simulink model "SF006A_TEstimn"  (R2013b)
settings: Solver=FixedStepDiscrete  StartTime=0.0  StopTime=1  FixedStep=0.1  RelTol=1e-3
values from neighbouring files (symbols this model uses):
  ARCHGLBPRM_100MILLISEC_SEC_F32 = DataDict.Constant    [SF006A_TEstimn_DataDict.m]
  ARCHGLBPRM_2MILLISEC_SEC_F32 = DataDict.Constant    [SF006A_TEstimn_DataDict.m]
  TEstimnAmbPwrMplr = DataDict.Calibration    [SF006A_TEstimn_DataDict.m]
  TEstimnAmbTSca = DataDict.Calibration    [SF006A_TEstimn_DataDict.m]
  TEstimnAssiMechAmbMplr = DataDict.Calibration    [SF006A_TEstimn_DataDict.m]
  TEstimnAssiMechCorrLim = DataDict.Calibration    [SF006A_TEstimn_DataDict.m]
  TEstimnAssiMechDampgSca = DataDict.Calibration    [SF006A_TEstimn_DataDict.m]
  TEstimnAssiMechDftT = DataDict.Calibration    [SF006A_TEstimn_DataDict.m]
  TEstimnAssiMechLLFilCoeffA1 = DataDict.Calibration    [SF006A_TEstimn_DataDict.m]
  TEstimnAssiMechLLFilCoeffB0 = DataDict.Calibration    [SF006A_TEstimn_DataDict.m]
  TEstimnAssiMechLLFilCoeffB1 = DataDict.Calibration    [SF006A_TEstimn_DataDict.m]
  TEstimnAssiMechSlew = DataDict.Calibration    [SF006A_TEstimn_DataDict.m]
  TESTIMNASSIMECHTHILIM_DEGCGRD_F32 = DataDict.Constant    [SF006A_TEstimn_DataDict.m]
  TESTIMNASSIMECHTLOLIM_DEGCGRD_F32 = DataDict.Constant    [SF006A_TEstimn_DataDict.m]
  TEstimnCorrnTAssiMech = DataDict.Calibration    [SF006A_TEstimn_DataDict.m]
  TEstimnCorrnTCu = DataDict.Calibration    [SF006A_TEstimn_DataDict.m]
  TEstimnCorrnTMag = DataDict.Calibration    [SF006A_TEstimn_DataDict.m]
  TEstimnCorrnTSi = DataDict.Calibration    [SF006A_TEstimn_DataDict.m]
  TEstimnCuAmbMplr = DataDict.Calibration    [SF006A_TEstimn_DataDict.m]
  TEstimnCuCorrnLim = DataDict.Calibration    [SF006A_TEstimn_DataDict.m]
  TEstimnCuLLFilCoeffA1 = DataDict.Calibration    [SF006A_TEstimn_DataDict.m]
  TEstimnCuLLFilCoeffB0 = DataDict.Calibration    [SF006A_TEstimn_DataDict.m]
  TEstimnCuLLFilCoeffB1 = DataDict.Calibration    [SF006A_TEstimn_DataDict.m]
  TEstimnEngTSca = DataDict.Calibration    [SF006A_TEstimn_DataDict.m]
  TESTIMNFETTHILIM_DEGCGRD_F32 = DataDict.Constant    [SF006A_TEstimn_DataDict.m]
  TESTIMNFETTLOLIM_DEGCGRD_F32 = DataDict.Constant    [SF006A_TEstimn_DataDict.m]
  TEstimnMagAmbMplr = DataDict.Calibration    [SF006A_TEstimn_DataDict.m]
  TEstimnMagCorrnLim = DataDict.Calibration    [SF006A_TEstimn_DataDict.m]
  TEstimnMagLLFilCoeffA1 = DataDict.Calibration    [SF006A_TEstimn_DataDict.m]
  TEstimnMagLLFilCoeffB0 = DataDict.Calibration    [SF006A_TEstimn_DataDict.m]
  TEstimnMagLLFilCoeffB1 = DataDict.Calibration    [SF006A_TEstimn_DataDict.m]
  TESTIMNMAGTHILIM_DEGCGRD_F32 = DataDict.Constant    [SF006A_TEstimn_DataDict.m]
  TESTIMNMAGTLOLIM_DEGCGRD_F32 = DataDict.Constant    [SF006A_TEstimn_DataDict.m]
  TEstimnSiAmbMplr = DataDict.Calibration    [SF006A_TEstimn_DataDict.m]
  TEstimnSiCorrnLim = DataDict.Calibration    [SF006A_TEstimn_DataDict.m]
  TEstimnSiLLFilCoeffA1 = DataDict.Calibration    [SF006A_TEstimn_DataDict.m]
  TEstimnSiLLFilCoeffB0 = DataDict.Calibration    [SF006A_TEstimn_DataDict.m]
  TEstimnSiLLFilCoeffB1 = DataDict.Calibration    [SF006A_TEstimn_DataDict.m]
  TEstimnWghtAvrgTDi = DataDict.Calibration    [SF006A_TEstimn_DataDict.m]
  TESTIMNWIDGTHILIM_DEGCGRD_F32 = DataDict.Constant    [SF006A_TEstimn_DataDict.m]
  TESTIMNWIDGTLOLIM_DEGCGRD_F32 = DataDict.Constant    [SF006A_TEstimn_DataDict.m]
undefined symbols (not defined in the file or in its folder): sigbuilder_block
libraries: NxtrLim x13, Fil x8, simulink x2
(part 2 of 3)

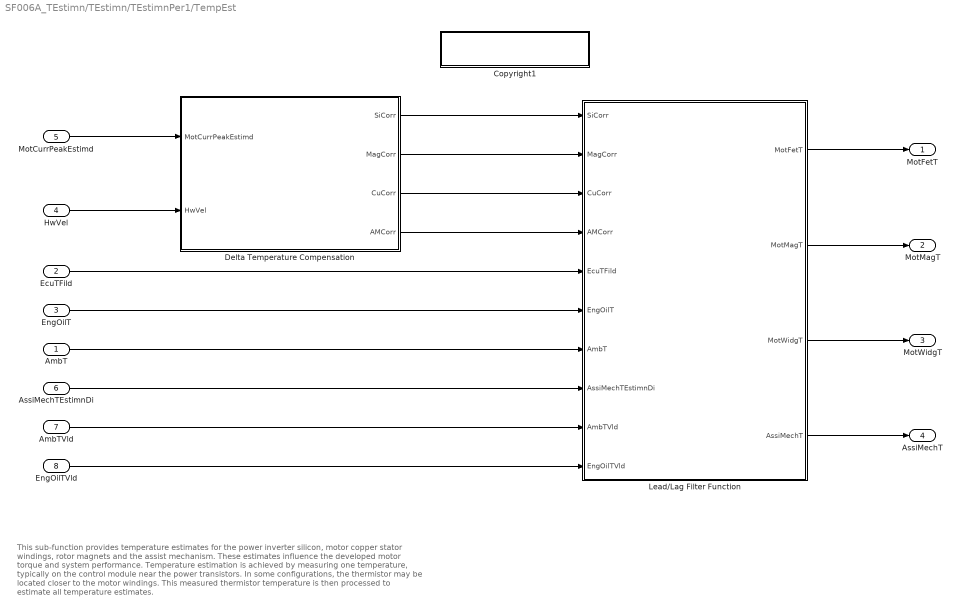
== system SF006A_TEstimn/TEstimn/TEstimnPer1/TempEst ==
  note: This sub-function provides temperature estimates for the power inverter silicon, motor copper stator windings, rotor magnets
      | and the assist mechanism. These estimates influence the developed motor torque and system performance.
      |
      | Temperature estimation is achieved by measuring one temperature, typically on the control module near the power transistors.
      | In some configurations, the thermistor may be located closer to the motor windings. This measured thermistor temperature is
      | then processed to estimate all temperature estimates.
  "AmbT " : Inport
  EcuTFild : Inport  Port=2
  "EngOilT " : Inport  Port=3
  "HwVel " : Inport  Port=4
  "MotCurrPeakEstimd " : Inport  Port=5
  AssiMechTEstimnDi : Inport  Port=6
  AmbTVld : Inport  Port=7
  EngOilTVld : Inport  Port=8
  Copyright1 : Subsystem  Description=|  RequirementInfo={} %GIDa_ed25a26e_86af_4b43_9ce6_79f2da1b6247  mask(Copyright Information){none=on}
      | Copyright info block.                                               
      |                                                                     
      | Place copyright information at the top of every subsystem in design.
      mask prompts: none "No parameters"
      mask help: Place copyright information at the top of every subsystem in design.
      mask Display:
      | NxtrConf = 'Nexteer Confidential';
      | 
      | sys = bdroot; %handle for the current model ("system")
      | first = get_param(sys,'Created');
      | if(isempty(first))
      |     first = datestr(now,'yyyy');
      | else
      |     first = first(end-3:end);  %year is last four digits
      | end
      | 
      | last = get_param(sys,'LastModifiedDate');
      | if isempty(last)
      |     last = datestr(now,'yyyy');
      | else
      |     last = last(end-3:end);
      | end
      | 
      | if strcmp(first,last)
      |     fprintf('%s\nCopyright  %s Nexteer',NxtrConf,first);
      | else
      |     fprintf('%s\n%s%s-%s Nexteer',NxtrConf,char(169),first,last);
      | end
  Delta Temperature Compensation : Subsystem  RequirementInfo={'linktype_rmi_doors' '0000a528 (/E-STEER Core/SubSystem Specifications/Application Functions/SF006A Temperature Estimation)' '#SF006A_128' 'true' 'REQ: SF006A_128' '' ; 'linktype_rmi_doors' '0000a528 (/E-STEER Core/SubSystem Specifications/Application Functions/SF006A Temperature Estimation)' '#SF006A_131' 'true' 'REQ: SF006A_131' '' ; 'linktype_rmi_doors' '0000a528 (/E-STEER Core/SubSystem Specifications/Application Functions/SF006A Temperature Estimation)' '#SF006A_145' 'true' 'REQ: SF006A_145' '' ; 'linktype_rmi_doors' '0000a528 (/E-STEER Core/SubSystem Specifications/Application Functions/SF006A Temperature Estimation)' '#SF006A_122' 'true' 'REQ: SF006A_122' '' } %GIDa_de2648f7_d571_4703_92ef_7b1b0dc2e478
  Lead/Lag Filter Function : Subsystem  RequirementInfo={'linktype_rmi_doors' '0000a528 (/E-STEER Core/SubSystem Specifications/Application Functions/SF006A Temperature Estimation)' '#SF006A_130' 'true' 'REQ: SF006A_130' '' ; 'linktype_rmi_doors' '0000a528 (/E-STEER Core/SubSystem Specifications/Application Functions/SF006A Temperature Estimation)' '#SF006A_132' 'true' 'REQ: SF006A_132' '' ; 'linktype_rmi_doors' '0000a528 (/E-STEER Core/SubSystem Specifications/Application Functions/SF006A Temperature Estimation)' '#SF006A_122' 'true' 'REQ: SF006A_122' '' ; 'linktype_rmi_doors' '0000a528 (/E-STEER Core/SubSystem Specifications/Application Functions/SF006A Temperature Estimation)' '#SF006A_170' 'true' 'REQ: SF006A_170' '' } %GIDa_ae028aaf_a7cd_4aef_92de_886aa640f764
  MotFetT : Outport
  MotMagT : Outport  Port=2
  MotWidgT : Outport  Port=3
  AssiMechT : Outport  Port=4
  wires:
  "MotCurrPeakEstimd "/1 -> Delta Temperature Compensation/1(MotCurrPeakEstimd)
  EcuTFild/1 -> Lead/Lag Filter Function/5(EcuTFild)
  Lead/Lag Filter Function/1(MotFetT) -> MotFetT/1
  Lead/Lag Filter Function/2(MotMagT) -> MotMagT/1
  Lead/Lag Filter Function/3(MotWidgT) -> MotWidgT/1
  Lead/Lag Filter Function/4(AssiMechT) -> AssiMechT/1
  "HwVel "/1 -> Delta Temperature Compensation/2(HwVel)
  "EngOilT "/1 -> Lead/Lag Filter Function/6("EngOilT ")
  "AmbT "/1 -> Lead/Lag Filter Function/7(AmbT)
  Delta Temperature Compensation/1(SiCorr) -> Lead/Lag Filter Function/1(SiCorr)
  Delta Temperature Compensation/2(MagCorr) -> Lead/Lag Filter Function/2(MagCorr)
  Delta Temperature Compensation/3(CuCorr) -> Lead/Lag Filter Function/3(CuCorr)
  Delta Temperature Compensation/4(AMCorr) -> Lead/Lag Filter Function/4(AMCorr)
  AssiMechTEstimnDi/1 -> Lead/Lag Filter Function/8(AssiMechTEstimnDi)
  EngOilTVld/1 -> Lead/Lag Filter Function/10(EngOilTVld)
  AmbTVld/1 -> Lead/Lag Filter Function/9(AmbTVld)

== system SF006A_TEstimn/TEstimn/TEstimnInit1/Assist Mechanism Temperature Initialization/AssistMechanismInitDisable ==
  EcuTFild : Inport
  Action Port : ActionPort  ActionType=else
  AssiMechT : Outport
  wires:
  EcuTFild/1 -> AssiMechT/1

== system SF006A_TEstimn/TEstimn/TEstimnInit1/Assist Mechanism Temperature Initialization/AssistMechanismInitEnable ==
  "EngOilT " : Inport
  AmbT : Inport  Port=2
  Action Port : ActionPort  ActionType=then
  Ambient Temperature Multiplier : Gain  Gain=TEstimnAmbTSca
      settings: AttributesFormatString=%<Gain>
  Engine Temperature Multiplier : Gain  Gain=TEstimnEngTSca
      settings: AttributesFormatString=%<Gain>
  Sum (4) : Sum  Inputs=+|+
  AssiMechT : Outport
  wires:
  "EngOilT "/1 -> Engine Temperature Multiplier/1
  Engine Temperature Multiplier/1 -> Sum (4)/1
  Ambient Temperature Multiplier/1 -> Sum (4)/2
  AmbT/1 -> Ambient Temperature Multiplier/1
  Sum (4)/1 -> AssiMechT/1

== system SF006A_TEstimn/TEstimn/TEstimnInit1/Assist Mechanism Temperature Initialization/Copyright1 ==

== system SF006A_TEstimn/TEstimn/TEstimnInit1/Assist Mechanism Temperature LeagLag Filter Initialization/Copyright1 ==

== system SF006A_TEstimn/TEstimn/TEstimnInit1/Motor Magnet Temperature Initialization/Copyright1 ==

== system SF006A_TEstimn/TEstimn/TEstimnInit1/Motor Magnet Temperature LeadLag Filter Initialization/Copyright1 ==

== system SF006A_TEstimn/TEstimn/TEstimnInit1/Motor Silicon Temperature Initialization/Copyright1 ==

== system SF006A_TEstimn/TEstimn/TEstimnInit1/Motor Silicon Temperature LeadLag Filter Initialization/Copyright1 ==

== system SF006A_TEstimn/TEstimn/TEstimnInit1/Motor Winding  Temperature Initialization /Copyright1 ==

== system SF006A_TEstimn/TEstimn/TEstimnInit1/Motor Winding  Temperature Lead Lag Initialization /Copyright1 ==

== system SF006A_TEstimn/TEstimn/TEstimnPer1/TempEst/Copyright1 ==

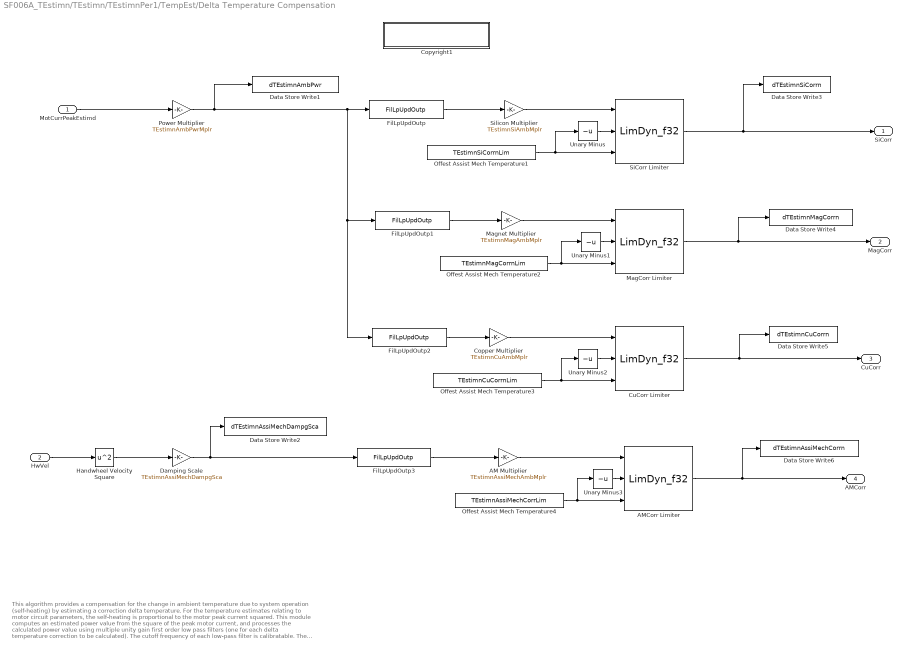
== system SF006A_TEstimn/TEstimn/TEstimnPer1/TempEst/Delta Temperature Compensation ==
  note: This algorithm provides a compensation for the change in ambient temperature due to system operation (self-heating) by estimating
      | a correction delta temperature.
      |
      | For the temperature estimates relating to motor circuit parameters, the self-heating is proportional to the motor peak current squared.
      | This module computes an estimated power value from the square of the peak motor current, and processes the calculated power value
      | using multiple unity gain first order low pass filters (one for each delta temperature correction to be calculated). The cutoff frequency of
      | each low-pass filter is calibratable. The output of each low pass filter is multiplied by a calibratable multiplier to appropriately scale the
      | result for each temperature estimate. The estimated correction temperature is also limited by a lower and upper bound.
      | For the assist mechanism temperature estimate, the self-heating is primarily due to energy dissipated due to system damping losses
      | which are proportional to the square of the rotational speed of the assist mechanism. The handwheel velocity is used to represent the
      | assist mechanism velocity. The handwheel velocity is squared and then scaled by a damping constant, and thereafter filtered through a
      | low pass filter with a calibratable frequency.
      |
      | Note that the state variables of all low pass filters must be initialized to zero at the beginning of each ignition cycle.
  MotCurrPeakEstimd : Inport
  HwVel : Inport  Port=2
  AM Multiplier : Gain  Gain=TEstimnAssiMechAmbMplr
      settings: AttributesFormatString=%<Gain>
  AMCorr Limiter : NxtrLim/LimDyn_f32
  Copper Multiplier : Gain  Gain=TEstimnCuAmbMplr
      settings: AttributesFormatString=%<Gain>
  Copyright1 : Subsystem  Description=|  RequirementInfo={} %GIDa_bd808200_6657_4ccc_9ad3_e79ac2c751ed  mask(Copyright Information){none=on}
      | Copyright info block.                                               
      |                                                                     
      | Place copyright information at the top of every subsystem in design.
      mask prompts: none "No parameters"
      mask help: Place copyright information at the top of every subsystem in design.
      mask Display:
      | NxtrConf = 'Nexteer Confidential';
      | 
      | sys = bdroot; %handle for the current model ("system")
      | first = get_param(sys,'Created');
      | if(isempty(first))
      |     first = datestr(now,'yyyy');
      | else
      |     first = first(end-3:end);  %year is last four digits
      | end
      | 
      | last = get_param(sys,'LastModifiedDate');
      | if isempty(last)
      |     last = datestr(now,'yyyy');
      | else
      |     last = last(end-3:end);
      | end
      | 
      | if strcmp(first,last)
      |     fprintf('%s\nCopyright  %s Nexteer',NxtrConf,first);
      | else
      |     fprintf('%s\n%s%s-%s Nexteer',NxtrConf,char(169),first,last);
      | end
  CuCorr Limiter : NxtrLim/LimDyn_f32
  Damping Scale : Gain  Gain=TEstimnAssiMechDampgSca  OutDataTypeStr=Inherit: Inherit via back propagation
      settings: AttributesFormatString=%<Gain>
  Data Store Write1 : DataStoreWrite  DataStoreName=dTEstimnAmbPwr
  Data Store Write2 : DataStoreWrite  DataStoreName=dTEstimnAssiMechDampgSca
  Data Store Write3 : DataStoreWrite  DataStoreName=dTEstimnSiCorrn
  Data Store Write4 : DataStoreWrite  DataStoreName=dTEstimnMagCorrn
  Data Store Write5 : DataStoreWrite  DataStoreName=dTEstimnCuCorrn
  Data Store Write6 : DataStoreWrite  DataStoreName=dTEstimnAssiMechCorrn
  FilLpUpdOutp : Fil/FilLpUpdOutp  StVar=SiFilLp
      settings: AttributesFormatString=StVar: %<StVar>
  FilLpUpdOutp1 : Fil/FilLpUpdOutp  StVar=MagFilLp
      settings: AttributesFormatString=StVar: %<StVar>
  FilLpUpdOutp2 : Fil/FilLpUpdOutp  StVar=CuFilLp
      settings: AttributesFormatString=StVar: %<StVar>
  FilLpUpdOutp3 : Fil/FilLpUpdOutp  StVar=AssiMechFilLp
      settings: AttributesFormatString=StVar: %<StVar>
  Handwheel Velocity Square : Math  Operator=square  OutDataTypeStr=Inherit: Inherit via back propagation  SaturateOnIntegerOverflow=on
  MagCorr Limiter : NxtrLim/LimDyn_f32
  Magnet Multiplier : Gain  Gain=TEstimnMagAmbMplr
      settings: AttributesFormatString=%<Gain>
  Offest Assist Mech Temperature1 : Constant  Value=TEstimnSiCorrnLim
  Offest Assist Mech Temperature2 : Constant  Value=TEstimnMagCorrnLim
  Offest Assist Mech Temperature3 : Constant  Value=TEstimnCuCorrnLim
  Offest Assist Mech Temperature4 : Constant  Value=TEstimnAssiMechCorrLim
  Power Multiplier : Gain  Gain=TEstimnAmbPwrMplr
      settings: AttributesFormatString=%<Gain>
  SiCorr Limiter : NxtrLim/LimDyn_f32
  Silicon Multiplier : Gain  Gain=TEstimnSiAmbMplr
      settings: AttributesFormatString=%<Gain>
  Unary Minus{,1..3} (4 alike) : UnaryMinus
  SiCorr : Outport
  MagCorr : Outport  Port=2
  CuCorr : Outport  Port=3
  AMCorr : Outport  Port=4
  wires:
  MotCurrPeakEstimd/1 -> Power Multiplier/1
  Silicon Multiplier/1 -> SiCorr Limiter/1
  Magnet Multiplier/1 -> MagCorr Limiter/1
  MagCorr Limiter/1 -> MagCorr/1, Data Store Write4/1
  Copper Multiplier/1 -> CuCorr Limiter/1
  AM Multiplier/1 -> AMCorr Limiter/1
  Damping Scale/1 -> Data Store Write2/1, FilLpUpdOutp3/1
  FilLpUpdOutp1/1 -> Magnet Multiplier/1
  Power Multiplier/1 -> Data Store Write1/1, FilLpUpdOutp2/1, FilLpUpdOutp1/1, FilLpUpdOutp/1
  FilLpUpdOutp/1 -> Silicon Multiplier/1
  FilLpUpdOutp2/1 -> Copper Multiplier/1
  FilLpUpdOutp3/1 -> AM Multiplier/1
  CuCorr Limiter/1 -> Data Store Write5/1, CuCorr/1
  Handwheel Velocity Square/1 -> Damping Scale/1
  HwVel/1 -> Handwheel Velocity Square/1
  Offest Assist Mech Temperature1/1 -> Unary Minus/1, SiCorr Limiter/3
  Unary Minus/1 -> SiCorr Limiter/2
  SiCorr Limiter/1 -> Data Store Write3/1, SiCorr/1
  Offest Assist Mech Temperature2/1 -> Unary Minus1/1, MagCorr Limiter/3
  Unary Minus1/1 -> MagCorr Limiter/2
  Offest Assist Mech Temperature3/1 -> Unary Minus2/1, CuCorr Limiter/3
  Unary Minus2/1 -> CuCorr Limiter/2
  Offest Assist Mech Temperature4/1 -> AMCorr Limiter/3, Unary Minus3/1
  Unary Minus3/1 -> AMCorr Limiter/2
  AMCorr Limiter/1 -> AMCorr/1, Data Store Write6/1

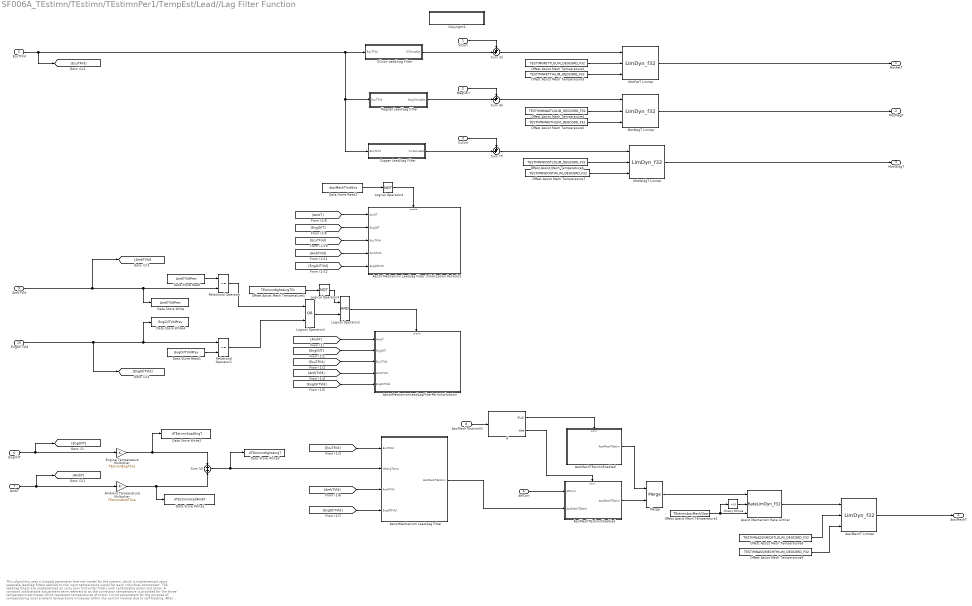
== system SF006A_TEstimn/TEstimn/TEstimnPer1/TempEst/Lead//Lag Filter Function ==
  note: This algorithm uses a lumped parameter thermal model for the system, which is implemented using separate lead/lag filters applied to the
      | input temperature signal for each individual component. The lead/lag filters are implemented as unity gain first-order filters with calibratable
      | poles and zeros.
      |
      | A constant calibratable adjustment term referred to as the correction temperature is provided for the three temperature estimates which represent
      | temperatures of motor circuit parameters for the purpose of compensating local ambient temperature increases within the control module
      | due to self-heating. After filtering the adjusted measured temperature, the corresponding correction term is added to the filter output to obtain
      | the final temperature estimate.
      | The Assist Mechanism temperature may be completely decoupled from the controller temperature and therefore the temperature estimate
      | filter does not use the measured controller temperature for an input. Two temperature inputs received from the vehicle serial communications
      | interface, namely the engine and ambient temperatures are used instead. Both of them are scaled separately and added, and this composite
      | temperature is used as the input to the lead/lag filter. Thereafter, the correction temperature is added to obtain the final estimate, and the rate
      | of change of the output is limited by a slew rate. The Assist Mechanism can be completely defeated using a serial communications message
      | if required.
      |
      | The exact details of the architecture as well as the method of initialization and reinitialization of each lead-lag flter is specified inside the
      | appropriate subsystems above.
  SiCorr : Inport
  MagCorr : Inport  Port=2
  CuCorr : Inport  Port=3
  AMCorr : Inport  Port=4
  EcuTFild : Inport  Port=5
  "EngOilT " : Inport  Port=6
  AmbT : Inport  Port=7
  AssiMechTEstimnDi : Inport  Port=8
  AmbTVld : Inport  Port=9
  EngOilTVld : Inport  Port=10
  Ambient Temperature Multiplier : Gain  Gain=TEstimnAmbTSca
      settings: AttributesFormatString=%<Gain>
  AssiMechT Limiter : NxtrLim/LimDyn_f32  RequirementInfo={'linktype_rmi_doors' '0000a528 (/E-STEER Core/SubSystem Specifications/Application Functions/SF006A Temperature Estimation)' '#SF006A_146' 'true' 'REQ: SF006A_146' '' } %GIDa_6c7b509c_1943_4e07_8eaa_8fab763417b2
  AssiMechTEstimnDisabled : Subsystem  RequirementInfo={'linktype_rmi_doors' '0000a528 (/E-STEER Core/SubSystem Specifications/Application Functions/SF006A Temperature Estimation)' '#SF006A_172' 'true' 'REQ: SF006A_172' '' } %GIDa_63efcaa1_2f18_430b_bd87_31b2ba6394f0  TreatAsAtomicUnit=on
  AssiMechTEstimnEnabled : Subsystem  RequirementInfo={'linktype_rmi_doors' '0000a528 (/E-STEER Core/SubSystem Specifications/Application Functions/SF006A Temperature Estimation)' '#SF006A_140' 'true' 'REQ: SF006A_140' '' ; 'linktype_rmi_doors' '0000a528 (/E-STEER Core/SubSystem Specifications/Application Functions/SF006A Temperature Estimation)' '#SF006A_172' 'true' 'REQ: SF006A_172' '' } %GIDa_baf7acd0_a9d7_4171_bbf7_6ce56e99201e  TreatAsAtomicUnit=on
  Assist Mechanism LeadLag Filter Initialization Periodic1 : Subsystem
  Assist Mechanism Rate Limiter : NxtrLim/RateLimDyn_f32  RequirementInfo={'linktype_rmi_doors' '0000a528 (/E-STEER Core/SubSystem Specifications/Application Functions/SF006A Temperature Estimation)' '#SF006A_159' 'true' 'REQ: SF006A_159' '' } %GIDa_cb60f311_8e3b_4de8_bd2f_2548d52e3f95  StVar=AssiMechTSlewLimPrev  Ts=ARCHGLBPRM_2MILLISEC_SEC_F32
      settings: AttributesFormatString=StVar: %<StVar>
  AssistMechanism Lead/Lag Filter : Subsystem  RequirementInfo={'linktype_rmi_doors' '0000a528 (/E-STEER Core/SubSystem Specifications/Application Functions/SF006A Temperature Estimation)' '#SF006A_135' 'true' 'REQ: SF006A_135' '' ; 'linktype_rmi_doors' '0000a528 (/E-STEER Core/SubSystem Specifications/Application Functions/SF006A Temperature Estimation)' '#SF006A_172' 'true' 'REQ: SF006A_172' '' } %GIDa_9c5c2d5a_035f_4761_9bec_ce6d38b05342
  AssistMechanismLeadLagFilterRe-Initialization : Subsystem  TreatAsAtomicUnit=on
  Copper Lead/Lag Filter : Subsystem  RequirementInfo={'linktype_rmi_doors' '0000a528 (/E-STEER Core/SubSystem Specifications/Application Functions/SF006A Temperature Estimation)' '#SF006A_171' 'true' 'REQ: SF006A_171' '' } %GIDa_b47124fe_ed06_4a6b_a9f5_ebcf66ffad42
  Copyright1 : Subsystem  Description=|  RequirementInfo={} %GIDa_98982cac_2d88_4b10_afa1_ae036335a444  mask(Copyright Information){none=on}
      | Copyright info block.                                               
      |                                                                     
      | Place copyright information at the top of every subsystem in design.
      mask prompts: none "No parameters"
      mask help: Place copyright information at the top of every subsystem in design.
      mask Display:
      | NxtrConf = 'Nexteer Confidential';
      | 
      | sys = bdroot; %handle for the current model ("system")
      | first = get_param(sys,'Created');
      | if(isempty(first))
      |     first = datestr(now,'yyyy');
      | else
      |     first = first(end-3:end);  %year is last four digits
      | end
      | 
      | last = get_param(sys,'LastModifiedDate');
      | if isempty(last)
      |     last = datestr(now,'yyyy');
      | else
      |     last = last(end-3:end);
      | end
      | 
      | if strcmp(first,last)
      |     fprintf('%s\nCopyright  %s Nexteer',NxtrConf,first);
      | else
      |     fprintf('%s\n%s%s-%s Nexteer',NxtrConf,char(169),first,last);
      | end
  Data Store Read : DataStoreRead  RequirementInfo={} %GIDa_9b0d40be_6666_4069_9c10_2ef51a624236  Priority=1  DataStoreName=AmbTVldPrev
      settings: AttributesFormatString="priority:  %<Priority>"
  Data Store Read1 : DataStoreRead  RequirementInfo={} %GIDa_19f52dbd_d2eb_4401_aae4_fbee21640a93  Priority=1  DataStoreName=EngOilTVldPrev
      settings: AttributesFormatString="priority:  %<Priority>"
  Data Store Read2 : DataStoreRead  DataStoreName=AssiMechTInitEna
  Data Store Write : DataStoreWrite  RequirementInfo={} %GIDa_1d441e6b_1fe9_4535_b703_6a16c57ac31c  Priority=2  DataStoreName=AmbTVldPrev
      settings: AttributesFormatString="priority:  %<Priority>"
  Data Store Write1 : DataStoreWrite  DataStoreName=dTEstimnScadAmbT
  Data Store Write2 : DataStoreWrite  DataStoreName=dTEstimnScadEngT
  Data Store Write3 : DataStoreWrite  DataStoreName=dTEstimnWghtAvrgT
  Data Store Write4 : DataStoreWrite  RequirementInfo={} %GIDa_a41cefac_a2e7_4b3f_b55c_d03ffcb12746  Priority=2  DataStoreName=EngOilTVldPrev
      settings: AttributesFormatString="priority:  %<Priority>"
  Engine Temperature Multiplier : Gain  Gain=TEstimnEngTSca
      settings: AttributesFormatString=%<Gain>
  If : If  IfExpression=u1
  Logical Operator1 : Logic  Operator=OR  AllPortsSameDT=off  OutDataTypeStr=boolean
  Logical Operator2 : Logic  AllPortsSameDT=off  OutDataTypeStr=boolean
  Logical Operator3 : Logic  Operator=NOT  AllPortsSameDT=off  OutDataTypeStr=boolean
  Logical Operator4 : Logic  Operator=NOT  AllPortsSameDT=off  OutDataTypeStr=boolean
  Magnet Lead/Lag Filter : Subsystem  RequirementInfo={'linktype_rmi_doors' '0000a528 (/E-STEER Core/SubSystem Specifications/Application Functions/SF006A Temperature Estimation)' '#SF006A_171' 'true' 'REQ: SF006A_171' '' } %GIDa_7145ecc5_8b30_4b7b_a3cc_c56f31d6ad47
  Merge : Merge
  MotFetT Limiter : NxtrLim/LimDyn_f32  RequirementInfo={'linktype_rmi_doors' '0000a528 (/E-STEER Core/SubSystem Specifications/Application Functions/SF006A Temperature Estimation)' '#SF006A_145' 'true' 'REQ: SF006A_145' '' ; 'linktype_rmi_doors' '0000a528 (/E-STEER Core/SubSystem Specifications/Application Functions/SF006A Temperature Estimation)' '#SF006A_147' 'true' 'REQ: SF006A_147' '' } %GIDa_13b78bce_d48c_485b_a8dd_8058a9fb1436
  MotMagT Limiter : NxtrLim/LimDyn_f32  RequirementInfo={'linktype_rmi_doors' '0000a528 (/E-STEER Core/SubSystem Specifications/Application Functions/SF006A Temperature Estimation)' '#SF006A_145' 'true' 'REQ: SF006A_145' '' ; 'linktype_rmi_doors' '0000a528 (/E-STEER Core/SubSystem Specifications/Application Functions/SF006A Temperature Estimation)' '#SF006A_147' 'true' 'REQ: SF006A_147' '' } %GIDa_60e1fd0e_a47d_43d3_86eb_3d2e6fed4866
  MotWidgT Limiter : NxtrLim/LimDyn_f32  RequirementInfo={'linktype_rmi_doors' '0000a528 (/E-STEER Core/SubSystem Specifications/Application Functions/SF006A Temperature Estimation)' '#SF006A_145' 'true' 'REQ: SF006A_145' '' ; 'linktype_rmi_doors' '0000a528 (/E-STEER Core/SubSystem Specifications/Application Functions/SF006A Temperature Estimation)' '#SF006A_147' 'true' 'REQ: SF006A_147' '' } %GIDa_2ee89f54_1f0f_4cc5_a14a_4440940f8ffc
  Offest Assist Mech Temperature1 : Constant  Value=TEstimnAssiMechSlew
  Offest Assist Mech Temperature2 : Constant  Value=TESTIMNFETTLOLIM_DEGCGRD_F32
  Offest Assist Mech Temperature3 : Constant  Value=TESTIMNFETTHILIM_DEGCGRD_F32
  Offest Assist Mech Temperature4 : Constant  Value=TESTIMNMAGTLOLIM_DEGCGRD_F32
  Offest Assist Mech Temperature5 : Constant  Value=TESTIMNMAGTHILIM_DEGCGRD_F32
  Offest Assist Mech Temperature6 : Constant  Value=TESTIMNWIDGTLOLIM_DEGCGRD_F32
  Offest Assist Mech Temperature7 : Constant  Value=TESTIMNWIDGTHILIM_DEGCGRD_F32
  Offest Assist Mech Temperature8 : Constant  Value=TESTIMNASSIMECHTLOLIM_DEGCGRD_F32
  Offest Assist Mech Temperature9 : Constant  Value=TESTIMNASSIMECHTHILIM_DEGCGRD_F32
  Offset Assist Mech Temperature1 : Constant  Value=TEstimnWghtAvrgTDi
  Relational Operator : RelationalOperator  Operator=~=  OutDataTypeStr=boolean
  Relational Operator1 : RelationalOperator  Operator=~=  OutDataTypeStr=boolean
  Silicon Lead/Lag Filter : Subsystem  RequirementInfo={'linktype_rmi_doors' '0000a528 (/E-STEER Core/SubSystem Specifications/Application Functions/SF006A Temperature Estimation)' '#SF006A_171' 'true' 'REQ: SF006A_171' '' } %GIDa_b6608b44_3176_48f0_b014_86631610bce1
  Sum (4) : Sum  Inputs=+|+
  Sum (5) : Sum  Inputs=++|
  Sum (6) : Sum  Inputs=++|
  Sum (7) : Sum  Inputs=++|
  Unary Minus : UnaryMinus
  MotFetT : Outport
  MotMagT : Outport  Port=2
  MotWidgT : Outport  Port=3
  AssiMechT : Outport  Port=4
  wires:
  EcuTFild/1 -> [EcuTFild], Silicon Lead/Lag Filter/1(EcuTFild), Copper Lead/Lag Filter/1(EcuTFild), Magnet Lead/Lag Filter/1(EcuTFild)
  MagCorr/1 -> Sum (6)/1
  CuCorr/1 -> Sum (7)/1
  SiCorr/1 -> Sum (5)/1
  Engine Temperature Multiplier/1 -> Sum (4)/1, Data Store Write2/1
  Ambient Temperature Multiplier/1 -> Data Store Write1/1, Sum (4)/2
  Copper Lead/Lag Filter/1(CuTempEst) -> Sum (7)/2
  Silicon Lead/Lag Filter/1(SiTempEst) -> Sum (5)/2
  AmbT/1 -> [AmbT], Ambient Temperature Multiplier/1
  Magnet Lead/Lag Filter/1(MagTempEst) -> Sum (6)/2
  "EngOilT "/1 -> [EngOilT], Engine Temperature Multiplier/1
  AMCorr/1 -> AssiMechTEstimnDisabled/1(AMCorr)
  AssiMechTEstimnDi/1 -> If/1
  AssiMechTEstimnEnabled/1(AssiMechTEstim) -> Merge/1
  AssiMechT Limiter/1 -> AssiMechT/1
  Sum (4)/1 -> AssistMechanism Lead/Lag Filter/2(WtAvgTemp), Data Store Write3/1
  Sum (5)/1 -> MotFetT Limiter/1
  MotFetT Limiter/1 -> MotFetT/1
  Sum (7)/1 -> MotWidgT Limiter/1
  MotWidgT Limiter/1 -> MotWidgT/1
  MotMagT Limiter/1 -> MotMagT/1
  Offest Assist Mech Temperature2/1 -> MotFetT Limiter/2
  Offest Assist Mech Temperature3/1 -> MotFetT Limiter/3
  Sum (6)/1 -> MotMagT Limiter/1
  Offest Assist Mech Temperature4/1 -> MotMagT Limiter/2
  Offest Assist Mech Temperature5/1 -> MotMagT Limiter/3
  Offest Assist Mech Temperature6/1 -> MotWidgT Limiter/2
  Offest Assist Mech Temperature7/1 -> MotWidgT Limiter/3
  Assist Mechanism Rate Limiter/1 -> AssiMechT Limiter/1
  Offest Assist Mech Temperature8/1 -> AssiMechT Limiter/2
  Offest Assist Mech Temperature9/1 -> AssiMechT Limiter/3
  Merge/1 -> Assist Mechanism Rate Limiter/1
  Offset Assist Mech Temperature1/1 -> Logical Operator3/1
  Logical Operator2/1 -> AssistMechanismLeadLagFilterRe-Initialization/Enable
  Logical Operator3/1 -> Logical Operator2/1
  [AmbT] -> AssistMechanismLeadLagFilterRe-Initialization/1(AmbT)
  [EcuTFild] -> AssistMechanismLeadLagFilterRe-Initialization/3(EcuTFild)
  [EngOilT] -> AssistMechanismLeadLagFilterRe-Initialization/2("EngOilT ")
  [EcuTFild] -> AssistMechanism Lead/Lag Filter/1(EcuTFild)
  AmbTVld/1 -> [AmbTVld], Relational Operator/2, Data Store Write/1
  EngOilTVld/1 -> Data Store Write4/1, Relational Operator1/1, [EngOilTVld]
  [AmbTVld] -> AssistMechanismLeadLagFilterRe-Initialization/4(AmbTVld)
  [EngOilTVld] -> AssistMechanismLeadLagFilterRe-Initialization/5(EngOilTVld)
  [AmbTVld] -> AssistMechanism Lead/Lag Filter/3(AmbTVld)
  [EngOilTVld] -> AssistMechanism Lead/Lag Filter/4(EngOilTVld)
  [EngOilTVld] -> Assist Mechanism LeadLag Filter Initialization Periodic1/5(EngOilTVld)
  [AmbT] -> Assist Mechanism LeadLag Filter Initialization Periodic1/1(AmbT)
  [EcuTFild] -> Assist Mechanism LeadLag Filter Initialization Periodic1/3(EcuTFild)
  [AmbTVld] -> Assist Mechanism LeadLag Filter Initialization Periodic1/4("AmbTVld ")
  [EngOilT] -> Assist Mechanism LeadLag Filter Initialization Periodic1/2(EngOilT)
  Data Store Read2/1 -> Logical Operator4/1
  AssiMechTEstimnDisabled/1(AssiMechTEstim) -> Merge/2
  If/1 -> AssiMechTEstimnEnabled/Action
  If/2 -> AssiMechTEstimnDisabled/Action
  AssistMechanism Lead/Lag Filter/1(AssiMechTEstimn) -> AssiMechTEstimnDisabled/2("AssiMechTEstim ")
  Unary Minus/1 -> Assist Mechanism Rate Limiter/2
  Offest Assist Mech Temperature1/1 -> Unary Minus/1, Assist Mechanism Rate Limiter/3
  Logical Operator1/1 -> Logical Operator2/2
  Relational Operator/1 -> Logical Operator1/1
  Relational Operator1/1 -> Logical Operator1/2
  Data Store Read/1 -> Relational Operator/1
  Data Store Read1/1 -> Relational Operator1/2
  Logical Operator4/1 -> Assist Mechanism LeadLag Filter Initialization Periodic1/Enable

== system SF006A_TEstimn/TEstimn/TEstimnPer1/TempEst/Delta Temperature Compensation/Copyright1 ==

== system SF006A_TEstimn/TEstimn/TEstimnPer1/TempEst/Lead//Lag Filter Function/AssiMechTEstimnDisabled ==
  AMCorr : Inport
  "AssiMechTEstim " : Inport  Port=2
  Action Port : ActionPort  ActionType=else
  Copyright1 : Subsystem  Description=|  RequirementInfo={} %GIDa_d7ebbfb5_0926_4f7a_b769_1281c8548293  mask(Copyright Information){none=on}
      | Copyright info block.                                               
      |                                                                     
      | Place copyright information at the top of every subsystem in design.
      mask prompts: none "No parameters"
      mask help: Place copyright information at the top of every subsystem in design.
      mask Display:
      | NxtrConf = 'Nexteer Confidential';
      | 
      | sys = bdroot; %handle for the current model ("system")
      | first = get_param(sys,'Created');
      | if(isempty(first))
      |     first = datestr(now,'yyyy');
      | else
      |     first = first(end-3:end);  %year is last four digits
      | end
      | 
      | last = get_param(sys,'LastModifiedDate');
      | if isempty(last)
      |     last = datestr(now,'yyyy');
      | else
      |     last = last(end-3:end);
      | end
      | 
      | if strcmp(first,last)
      |     fprintf('%s\nCopyright  %s Nexteer',NxtrConf,first);
      | else
      |     fprintf('%s\n%s%s-%s Nexteer',NxtrConf,char(169),first,last);
      | end
  Data Store Write2 : DataStoreWrite  DataStoreName=dTEstimnAssiMechFil
  Sum (9) : Sum  Inputs=++|
  AssiMechTEstim : Outport
  wires:
  AMCorr/1 -> Sum (9)/1
  "AssiMechTEstim "/1 -> Sum (9)/2
  Sum (9)/1 -> Data Store Write2/1, AssiMechTEstim/1

== system SF006A_TEstimn/TEstimn/TEstimnPer1/TempEst/Lead//Lag Filter Function/AssiMechTEstimnEnabled ==
  Action Port : ActionPort  ActionType=then
  Copyright1 : Subsystem  Description=|  RequirementInfo={} %GIDa_b35a3d50_9030_47a1_913f_f1540f527605  mask(Copyright Information){none=on}
      | Copyright info block.                                               
      |                                                                     
      | Place copyright information at the top of every subsystem in design.
      mask prompts: none "No parameters"
      mask help: Place copyright information at the top of every subsystem in design.
      mask Display:
      | NxtrConf = 'Nexteer Confidential';
      | 
      | sys = bdroot; %handle for the current model ("system")
      | first = get_param(sys,'Created');
      | if(isempty(first))
      |     first = datestr(now,'yyyy');
      | else
      |     first = first(end-3:end);  %year is last four digits
      | end
      | 
      | last = get_param(sys,'LastModifiedDate');
      | if isempty(last)
      |     last = datestr(now,'yyyy');
      | else
      |     last = last(end-3:end);
      | end
      | 
      | if strcmp(first,last)
      |     fprintf('%s\nCopyright  %s Nexteer',NxtrConf,first);
      | else
      |     fprintf('%s\n%s%s-%s Nexteer',NxtrConf,char(169),first,last);
      | end
  Offest Assist Mech Temperature1 : Constant  Value=TEstimnAssiMechDftT
  AssiMechTEstim : Outport
  wires:
  Offest Assist Mech Temperature1/1 -> AssiMechTEstim/1

== system SF006A_TEstimn/TEstimn/TEstimnPer1/TempEst/Lead//Lag Filter Function/Assist Mechanism LeadLag Filter Initialization Periodic1 ==
  AmbT : Inport
  EngOilT : Inport  Port=2
  EcuTFild : Inport  Port=3
  "AmbTVld " : Inport  Port=4
  EngOilTVld : Inport  RequirementInfo={} %GIDa_14f17b2c_6b8b_460b_94dc_86ca5086ad22  Port=5
  Enable : EnablePort
  AssistMechanismInitDisable : Subsystem
  AssistMechanismInitEnable : Subsystem
  Copyright1 : Subsystem  Description=|  RequirementInfo={} %GIDa_df85eb69_2758_4231_85c8_da117ef3c433  mask(Copyright Information){none=on}
      | Copyright info block.                                               
      |                                                                     
      | Place copyright information at the top of every subsystem in design.
      mask prompts: none "No parameters"
      mask help: Place copyright information at the top of every subsystem in design.
      mask Display:
      | NxtrConf = 'Nexteer Confidential';
      | 
      | sys = bdroot; %handle for the current model ("system")
      | first = get_param(sys,'Created');
      | if(isempty(first))
      |     first = datestr(now,'yyyy');
      | else
      |     first = first(end-3:end);  %year is last four digits
      | end
      | 
      | last = get_param(sys,'LastModifiedDate');
      | if isempty(last)
      |     last = datestr(now,'yyyy');
      | else
      |     last = last(end-3:end);
      | end
      | 
      | if strcmp(first,last)
      |     fprintf('%s\nCopyright  %s Nexteer',NxtrConf,first);
      | else
      |     fprintf('%s\n%s%s-%s Nexteer',NxtrConf,char(169),first,last);
      | end
  Data Store Write4 : DataStoreWrite  DataStoreName=AssiMechTInitEna
  If1 : If  IfExpression=u1
  Logical Operator : Logic  Operator=NOT  AllPortsSameDT=off  OutDataTypeStr=boolean
  Logical Operator4 : Logic  Inputs=3  AllPortsSameDT=off  OutDataTypeStr=boolean
  Offset Assist Mech Temperature2 : Constant  Value=TEstimnWghtAvrgTDi
  Zero : Constant  OutDataTypeStr=boolean
  wires:
  AmbT/1 -> AssistMechanismInitEnable/2(AmbT)
  EngOilTVld/1 -> Logical Operator4/3
  "AmbTVld "/1 -> Logical Operator4/2
  EcuTFild/1 -> AssistMechanismInitDisable/1(EcuTFild)
  Logical Operator4/1 -> If1/1
  EngOilT/1 -> AssistMechanismInitEnable/1("EngOilT ")
  Zero/1 -> Data Store Write4/1
  If1/1 -> AssistMechanismInitEnable/Action
  If1/2 -> AssistMechanismInitDisable/Action
  Logical Operator/1 -> Logical Operator4/1
  Offset Assist Mech Temperature2/1 -> Logical Operator/1

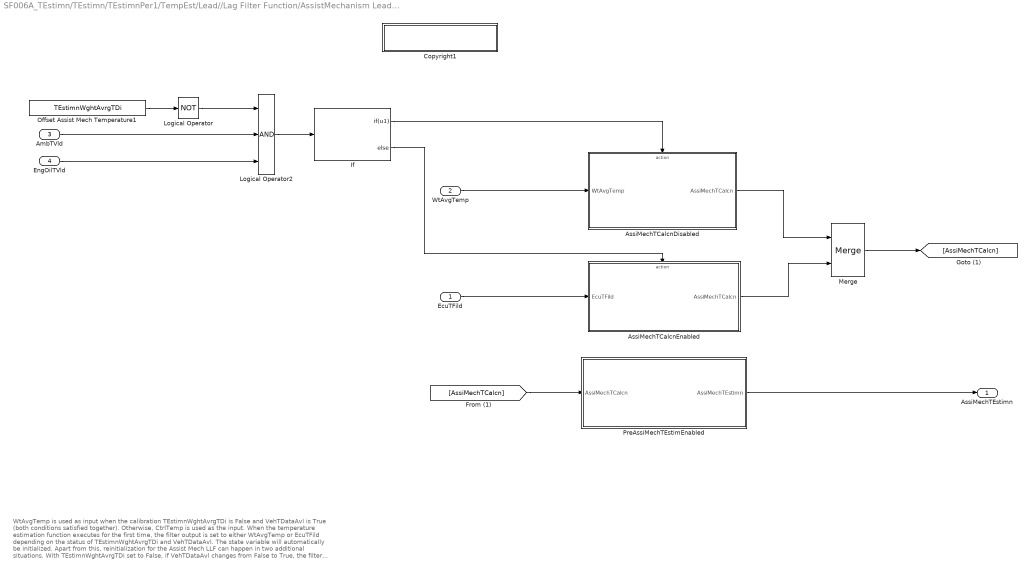
== system SF006A_TEstimn/TEstimn/TEstimnPer1/TempEst/Lead//Lag Filter Function/AssistMechanism Lead//Lag Filter ==
  note: WtAvgTemp is used as input when the calibration TEstimnWghtAvrgTDi is False and VehTDataAvl
      | is True (both conditions satisfied together). Otherwise, CtrlTemp is used as the input.
      |
      | When the temperature estimation function executes for the first time, the filter output is set to either WtAvgTemp
      | or EcuTFild depending on the status of TEstimnWghtAvrgTDi and VehTDataAvl. The state variable will
      | automatically be initialized. Apart from this, reinitialization for the Assist Mech LLF can happen in two additional
      | situations. With TEstimnWghtAvrgTDi set to False, if VehTDataAvl changes from False to True, the filter
      | output is set to WtAvgTemp. If VehTDataAvl changes from True to False, the filter output is set to
      | EcuTFild. In either of these cases, the state variable will automatically be initialized.
      |
      | The initialization scheme can be mathematically expressed as follows,
      | y(0) = CtrlTemp;
      | x(0) = A1*y(0) + B1*u(0);
      | where y = output, x = state variable, u = input
      |
      | The general equation for the n-th time-step will be,
      | y(n) = x(n-1) + B0*u(n);
      | x(n) = A1*y(n-1) + B1*u(n-1);
      |
      | Note that the filter needs to be re-initialized using the specified method at the beginning of each ignition cycle.
  EcuTFild : Inport
  WtAvgTemp : Inport  Port=2
  AmbTVld : Inport  Port=3
  EngOilTVld : Inport  Port=4
  AssiMechTCalcnDisabled : Subsystem  TreatAsAtomicUnit=on
  AssiMechTCalcnEnabled : Subsystem  TreatAsAtomicUnit=on
  Copyright1 : Subsystem  Description=|  RequirementInfo={} %GIDa_0cab8def_7a72_4ada_8d27_0185839ed81e  mask(Copyright Information){none=on}
      | Copyright info block.                                               
      |                                                                     
      | Place copyright information at the top of every subsystem in design.
      mask prompts: none "No parameters"
      mask help: Place copyright information at the top of every subsystem in design.
      mask Display:
      | NxtrConf = 'Nexteer Confidential';
      | 
      | sys = bdroot; %handle for the current model ("system")
      | first = get_param(sys,'Created');
      | if(isempty(first))
      |     first = datestr(now,'yyyy');
      | else
      |     first = first(end-3:end);  %year is last four digits
      | end
      | 
      | last = get_param(sys,'LastModifiedDate');
      | if isempty(last)
      |     last = datestr(now,'yyyy');
      | else
      |     last = last(end-3:end);
      | end
      | 
      | if strcmp(first,last)
      |     fprintf('%s\nCopyright  %s Nexteer',NxtrConf,first);
      | else
      |     fprintf('%s\n%s%s-%s Nexteer',NxtrConf,char(169),first,last);
      | end
  If : If  IfExpression=u1
  Logical Operator : Logic  Operator=NOT  AllPortsSameDT=off  OutDataTypeStr=boolean
  Logical Operator2 : Logic  Inputs=3  AllPortsSameDT=off  OutDataTypeStr=boolean
  Merge : Merge
  Offset Assist Mech Temperature1 : Constant  Value=TEstimnWghtAvrgTDi
  PreAssiMechTEstimEnabled : Subsystem  TreatAsAtomicUnit=on
  AssiMechTEstimn : Outport
  wires:
  EcuTFild/1 -> AssiMechTCalcnEnabled/1(EcuTFild)
  Logical Operator2/1 -> If/1
  Merge/1 -> [AssiMechTCalcn]
  Offset Assist Mech Temperature1/1 -> Logical Operator/1
  WtAvgTemp/1 -> AssiMechTCalcnDisabled/1(WtAvgTemp)
  [AssiMechTCalcn] -> PreAssiMechTEstimEnabled/1("AssiMechTCalcn ")
  Logical Operator/1 -> Logical Operator2/1
  AssiMechTCalcnDisabled/1(AssiMechTCalcn) -> Merge/1
  AssiMechTCalcnEnabled/1("AssiMechTCalcn ") -> Merge/2
  If/1 -> AssiMechTCalcnDisabled/Action
  If/2 -> AssiMechTCalcnEnabled/Action
  EngOilTVld/1 -> Logical Operator2/3
  AmbTVld/1 -> Logical Operator2/2
  PreAssiMechTEstimEnabled/1(AssiMechTEstimn) -> AssiMechTEstimn/1

== system SF006A_TEstimn/TEstimn/TEstimnPer1/TempEst/Lead//Lag Filter Function/AssistMechanismLeadLagFilterRe-Initialization ==
  AmbT : Inport
  "EngOilT " : Inport  Port=2
  EcuTFild : Inport  Port=3
  AmbTVld : Inport  Port=4
  EngOilTVld : Inport  Port=5
  Enable : EnablePort
  AssistMechanismInitDisable : Subsystem
  AssistMechanismInitEnable : Subsystem
  Copyright1 : Subsystem  Description=|  RequirementInfo={} %GIDa_a3fd27a8_0ee1_4cbe_aea6_761af5699832  mask(Copyright Information){none=on}
      | Copyright info block.                                               
      |                                                                     
      | Place copyright information at the top of every subsystem in design.
      mask prompts: none "No parameters"
      mask help: Place copyright information at the top of every subsystem in design.
      mask Display:
      | NxtrConf = 'Nexteer Confidential';
      | 
      | sys = bdroot; %handle for the current model ("system")
      | first = get_param(sys,'Created');
      | if(isempty(first))
      |     first = datestr(now,'yyyy');
      | else
      |     first = first(end-3:end);  %year is last four digits
      | end
      | 
      | last = get_param(sys,'LastModifiedDate');
      | if isempty(last)
      |     last = datestr(now,'yyyy');
      | else
      |     last = last(end-3:end);
      | end
      | 
      | if strcmp(first,last)
      |     fprintf('%s\nCopyright  %s Nexteer',NxtrConf,first);
      | else
      |     fprintf('%s\n%s%s-%s Nexteer',NxtrConf,char(169),first,last);
      | end
  If : If  IfExpression=u1
  Logical Operator1 : Logic  AllPortsSameDT=off  OutDataTypeStr=boolean
  wires:
  EcuTFild/1 -> AssistMechanismInitDisable/1(EcuTFild)
  "EngOilT "/1 -> AssistMechanismInitEnable/1("EngOilT ")
  AmbT/1 -> AssistMechanismInitEnable/2(AmbT)
  If/1 -> AssistMechanismInitEnable/Action
  If/2 -> AssistMechanismInitDisable/Action
  Logical Operator1/1 -> If/1
  EngOilTVld/1 -> Logical Operator1/2
  AmbTVld/1 -> Logical Operator1/1

== system SF006A_TEstimn/TEstimn/TEstimnPer1/TempEst/Lead//Lag Filter Function/Copper Lead//Lag Filter ==
  note: When the Temperature Estimation function executes for the first time, the filter output
      | is set to CtrlTemp. The state variable will automatically be initialized.
      |
      | The initialization scheme can be mathematically expressed as follows,
      | y(0) = CtrlTemp;
      | x(0) = A1*y(0) + B1*u(0);
      | where y = output, x = state variable, u = input
      |
      | The general equation for the n-th time-step will be,
      | y(n) = x(n-1) + B0*u(n);
      | x(n) = A1*y(n-1) + B1*u(n-1);
      |
      | Note that if the filter output is initialized (to zero) when the value of CtrlTemp is not stable,
      | the state variable will get initialized to an incorrect value, and will result in grossly incorrect
      | temperature estimates.
      |
      | Note that the filter needs to be re-initialized using the specified method at the beginning of
      | each ignition cycle.
  EcuTFild : Inport
  Copper Lead Lag Filter A1 : Constant  Value=TEstimnCuLLFilCoeffA1
  Copper Lead Lag Filter B0 : Constant  Value=TEstimnCuLLFilCoeffB0
  Copper Lead Lag Filter B2 : Constant  Value=TEstimnCuLLFilCoeffB1
  Copyright1 : Subsystem  Description=|  RequirementInfo={} %GIDa_55e7c6e6_812f_4d94_8f33_617c6b0e9d3d  mask(Copyright Information){none=on}
      | Copyright info block.                                               
      |                                                                     
      | Place copyright information at the top of every subsystem in design.
      mask prompts: none "No parameters"
      mask help: Place copyright information at the top of every subsystem in design.
      mask Display:
      | NxtrConf = 'Nexteer Confidential';
      | 
      | sys = bdroot; %handle for the current model ("system")
      | first = get_param(sys,'Created');
      | if(isempty(first))
      |     first = datestr(now,'yyyy');
      | else
      |     first = first(end-3:end);  %year is last four digits
      | end
      | 
      | last = get_param(sys,'LastModifiedDate');
      | if isempty(last)
      |     last = datestr(now,'yyyy');
      | else
      |     last = last(end-3:end);
      | end
      | 
      | if strcmp(first,last)
      |     fprintf('%s\nCopyright  %s Nexteer',NxtrConf,first);
      | else
      |     fprintf('%s\n%s%s-%s Nexteer',NxtrConf,char(169),first,last);
      | end
  Data Store Read : DataStoreRead  DataStoreName=CuTEstimnPrev
  Data Store Write1 : DataStoreWrite  DataStoreName=CuTEstimnPrev
  Offset Copper Temperature : Constant  Value=TEstimnCorrnTCu
  Product (1)1 : Product  RndMeth=Zero
  Product (2) : Product  RndMeth=Zero
  Product (3) : Product  RndMeth=Zero
  Sum (2)1 : Sum  Inputs=++|
  Sum (3)3 : Sum  Inputs=++|
  Sum (3)4 : Sum  Inputs=++|
  CuTempEst : Outport
  wires:
  Data Store Read/1 -> Sum (2)1/1
  Offset Copper Temperature/1 -> Sum (3)3/1
  Sum (3)3/1 -> Product (2)/2, Product (1)1/2
  Sum (2)1/1 -> CuTempEst/1, Product (3)/1
  Copper Lead Lag Filter A1/1 -> Product (3)/2
  Copper Lead Lag Filter B2/1 -> Product (2)/1
  Product (2)/1 -> Sum (3)4/2
  Product (3)/1 -> Sum (3)4/1
  Copper Lead Lag Filter B0/1 -> Product (1)1/1
  Sum (3)4/1 -> Data Store Write1/1
  Product (1)1/1 -> Sum (2)1/2
  EcuTFild/1 -> Sum (3)3/2

== system SF006A_TEstimn/TEstimn/TEstimnPer1/TempEst/Lead//Lag Filter Function/Copyright1 ==

== system SF006A_TEstimn/TEstimn/TEstimnPer1/TempEst/Lead//Lag Filter Function/Magnet Lead//Lag Filter ==
  note: When the Temperature Estimation function executes for the first time, the filter output
      | is set to CtrlTemp. The state variable will automatically be initialized.
      |
      | The initialization scheme can be mathematically expressed as follows,
      | y(0) = CtrlTemp;
      | x(0) = A1*y(0) + B1*u(0);
      | where y = output, x = state variable, u = input
      |
      | The general equation for the n-th time-step will be,
      | y(n) = x(n-1) + B0*u(n);
      | x(n) = A1*y(n-1) + B1*u(n-1);
      |
      | Note that if the filter output is initialized (to zero) when the value of CtrlTemp is not stable,
      | the state variable will get initialized to an incorrect value, and will result in grossly incorrect
      | temperature estimates.
      |
      | Note that the filter needs to be re-initialized using the specified method at the beginning of
      | each ignition cycle.
  EcuTFild : Inport
  Copyright1 : Subsystem  Description=|  RequirementInfo={} %GIDa_333c0fd3_841d_4587_a7c4_0b48229b0150  mask(Copyright Information){none=on}
      | Copyright info block.                                               
      |                                                                     
      | Place copyright information at the top of every subsystem in design.
      mask prompts: none "No parameters"
      mask help: Place copyright information at the top of every subsystem in design.
      mask Display:
      | NxtrConf = 'Nexteer Confidential';
      | 
      | sys = bdroot; %handle for the current model ("system")
      | first = get_param(sys,'Created');
      | if(isempty(first))
      |     first = datestr(now,'yyyy');
      | else
      |     first = first(end-3:end);  %year is last four digits
      | end
      | 
      | last = get_param(sys,'LastModifiedDate');
      | if isempty(last)
      |     last = datestr(now,'yyyy');
      | else
      |     last = last(end-3:end);
      | end
      | 
      | if strcmp(first,last)
      |     fprintf('%s\nCopyright  %s Nexteer',NxtrConf,first);
      | else
      |     fprintf('%s\n%s%s-%s Nexteer',NxtrConf,char(169),first,last);
      | end
  Data Store Read : DataStoreRead  DataStoreName=MagTEstimnPrev
  Data Store Write1 : DataStoreWrite  DataStoreName=MagTEstimnPrev
  Magnet Lead Lag Filter A1 : Constant  Value=TEstimnMagLLFilCoeffA1
  Magnet Lead Lag Filter B0 : Constant  Value=TEstimnMagLLFilCoeffB0
  Magnet Lead Lag Filter B1 : Constant  Value=TEstimnMagLLFilCoeffB1
  Offset Copper Temperature1 : Constant  Value=TEstimnCorrnTMag
  Product (1)1 : Product  RndMeth=Zero
  Product (2) : Product  RndMeth=Zero
  Product (3) : Product  RndMeth=Zero
  Sum (2)1 : Sum  Inputs=++|
  Sum (3)3 : Sum  Inputs=++|
  Sum (3)4 : Sum  Inputs=++|
  MagTempEst : Outport
  wires:
  Data Store Read/1 -> Sum (2)1/1
  Offset Copper Temperature1/1 -> Sum (3)3/1
  Sum (3)3/1 -> Product (2)/2, Product (1)1/2
  Sum (2)1/1 -> MagTempEst/1, Product (3)/1
  Magnet Lead Lag Filter A1/1 -> Product (3)/2
  Magnet Lead Lag Filter B1/1 -> Product (2)/1
  Product (2)/1 -> Sum (3)4/2
  Product (3)/1 -> Sum (3)4/1
  Magnet Lead Lag Filter B0/1 -> Product (1)1/1
  Sum (3)4/1 -> Data Store Write1/1
  Product (1)1/1 -> Sum (2)1/2
  EcuTFild/1 -> Sum (3)3/2
